simulink subsystem "Joystick_Input_To_Swerve_Drive_sub"  (R2023b)
settings: Solver=VariableStepAuto  StartTime=0.0  StopTime=10.0  RelTol=1e-3
undefined symbols (not defined in the file): AT_XY_Control_Gain, AT_Yaw_Control_Gain, Boost_Trigger_High_Speed, Boost_Trigger_Low_Speed, Steering_Abs_Deadband_Range, Steering_Mod_Drv_in, Steering_Mod_Drv_out, Steering_Mod_Str_Rel_in, Steering_Mod_Str_Rel_out, Steering_Relative_Gain, Steering_Twist_Gain, Translation_Twist_Gain
libraries: simulink x14, hdlsllib x5, Controls_Components_lib x1
settings Model: Creator=ander  LastModifiedBy=FIRSTMentor

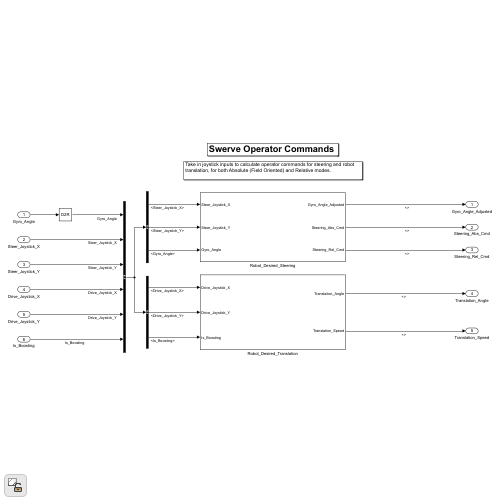
[thumbnail: Simulink's stored preview of the top-level diagram]
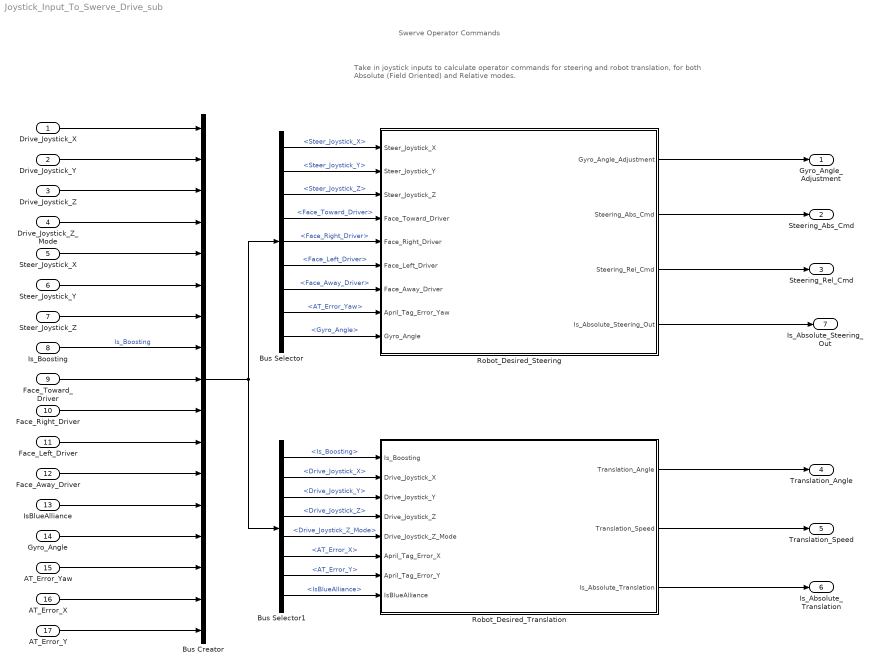
== system Joystick_Input_To_Swerve_Drive_sub ==
  note: Swerve Operator Commands
  note: Take in joystick inputs to calculate operator commands for steering and robot translation, for both Absolute (Field Oriented) and Relative modes.
  Drive_Joystick_X : Inport
  Drive_Joystick_Y : Inport  Port=2
  Drive_Joystick_Z : Inport  Port=3
  Drive_Joystick_Z_Mode : Inport  Port=4
  Steer_Joystick_X : Inport  Port=5
  Steer_Joystick_Y : Inport  Port=6
  Steer_Joystick_Z : Inport  Port=7
  Is_Boosting : Inport  Port=8
  Face_Toward_Driver : Inport  Port=9
  Face_Right_Driver : Inport  Port=10
  Face_Left_Driver : Inport  Port=11
  Face_Away_Driver : Inport  Port=12
  IsBlueAlliance : Inport  Port=13
  Gyro_Angle : Inport  Port=14
  AT_Error_Yaw : Inport  Port=15
  AT_Error_X : Inport  Port=16
  AT_Error_Y : Inport  Port=17
  Bus Creator : BusCreator  Inputs=17
  Bus Selector : BusSelector  OutputSignals=Steer_Joystick_X,Steer_Joystick_Y,Steer_Joystick_Z,Face_Toward_Driver,Face_Right_Driver,Face_Left_Driver,Face_Away_Driver,AT_Error_Yaw,Gyro_Angle
  Bus Selector1 : BusSelector  OutputSignals=Is_Boosting,Drive_Joystick_X,Drive_Joystick_Y,Drive_Joystick_Z,Drive_Joystick_Z_Mode,AT_Error_X,AT_Error_Y,IsBlueAlliance
  Robot_Desired_Steering : Subsystem
  Robot_Desired_Translation : Subsystem
  Gyro_Angle_Adjustment : Outport
  Steering_Abs_Cmd : Outport  Port=2
  Steering_Rel_Cmd : Outport  Port=3
  Translation_Angle : Outport  Port=4
  Translation_Speed : Outport  Port=5
  Is_Absolute_Translation : Outport  Port=6
  Is_Absolute_Steering_Out : Outport  Port=7
  wires:
  Robot_Desired_Steering/4(Is_Absolute_Steering_Out) -> Is_Absolute_Steering_Out/1
  Bus Selector1/5 -> Robot_Desired_Translation/5(Drive_Joystick_Z_Mode)  "<Drive_Joystick_Z_Mode>"
  Drive_Joystick_Z_Mode/1 -> Bus Creator/4
  Bus Selector1/7 -> Robot_Desired_Translation/7(April_Tag_Error_Y)  "<AT_Error_Y>"
  Bus Selector1/6 -> Robot_Desired_Translation/6(April_Tag_Error_X)  "<AT_Error_X>"
  Bus Selector/8 -> Robot_Desired_Steering/8(April_Tag_Error_Yaw)  "<AT_Error_Yaw>"
  Robot_Desired_Translation/3(Is_Absolute_Translation) -> Is_Absolute_Translation/1
  Bus Selector1/4 -> Robot_Desired_Translation/4(Drive_Joystick_Z)  "<Drive_Joystick_Z>"
  Bus Selector1/1 -> Robot_Desired_Translation/1(Is_Boosting)  "<Is_Boosting>"
  Robot_Desired_Steering/3(Steering_Rel_Cmd) -> Steering_Rel_Cmd/1
  Robot_Desired_Steering/2(Steering_Abs_Cmd) -> Steering_Abs_Cmd/1
  Robot_Desired_Steering/1(Gyro_Angle_Adjustment) -> Gyro_Angle_Adjustment/1
  Bus Selector/2 -> Robot_Desired_Steering/2(Steer_Joystick_Y)  "<Steer_Joystick_Y>"
  Bus Selector/1 -> Robot_Desired_Steering/1(Steer_Joystick_X)  "<Steer_Joystick_X>"
  Robot_Desired_Translation/1(Translation_Angle) -> Translation_Angle/1
  Robot_Desired_Translation/2(Translation_Speed) -> Translation_Speed/1
  Bus Creator/1 -> Bus Selector/1, Bus Selector1/1
  Bus Selector1/3 -> Robot_Desired_Translation/3(Drive_Joystick_Y)  "<Drive_Joystick_Y>"
  Bus Selector1/2 -> Robot_Desired_Translation/2(Drive_Joystick_X)  "<Drive_Joystick_X>"
  Drive_Joystick_X/1 -> Bus Creator/1
  Drive_Joystick_Z/1 -> Bus Creator/3
  Steer_Joystick_Y/1 -> Bus Creator/6
  Drive_Joystick_Y/1 -> Bus Creator/2
  Steer_Joystick_X/1 -> Bus Creator/5
  Steer_Joystick_Z/1 -> Bus Creator/7
  Face_Toward_Driver/1 -> Bus Creator/9
  Face_Right_Driver/1 -> Bus Creator/10
  Face_Left_Driver/1 -> Bus Creator/11
  Face_Away_Driver/1 -> Bus Creator/12
  Is_Boosting/1 -> Bus Creator/8  "Is_Boosting"
  Bus Selector/4 -> Robot_Desired_Steering/4(Face_Toward_Driver)  "<Face_Toward_Driver>"
  Bus Selector/3 -> Robot_Desired_Steering/3(Steer_Joystick_Z)  "<Steer_Joystick_Z>"
  Bus Selector/5 -> Robot_Desired_Steering/5(Face_Right_Driver)  "<Face_Right_Driver>"
  Bus Selector/6 -> Robot_Desired_Steering/6(Face_Left_Driver)  "<Face_Left_Driver>"
  Bus Selector/7 -> Robot_Desired_Steering/7(Face_Away_Driver)  "<Face_Away_Driver>"
  IsBlueAlliance/1 -> Bus Creator/13
  AT_Error_Yaw/1 -> Bus Creator/15
  AT_Error_X/1 -> Bus Creator/16
  AT_Error_Y/1 -> Bus Creator/17
  Bus Selector1/8 -> Robot_Desired_Translation/8(IsBlueAlliance)  "<IsBlueAlliance>"
  Gyro_Angle/1 -> Bus Creator/14
  Bus Selector/9 -> Robot_Desired_Steering/9(Gyro_Angle)  "<Gyro_Angle>"

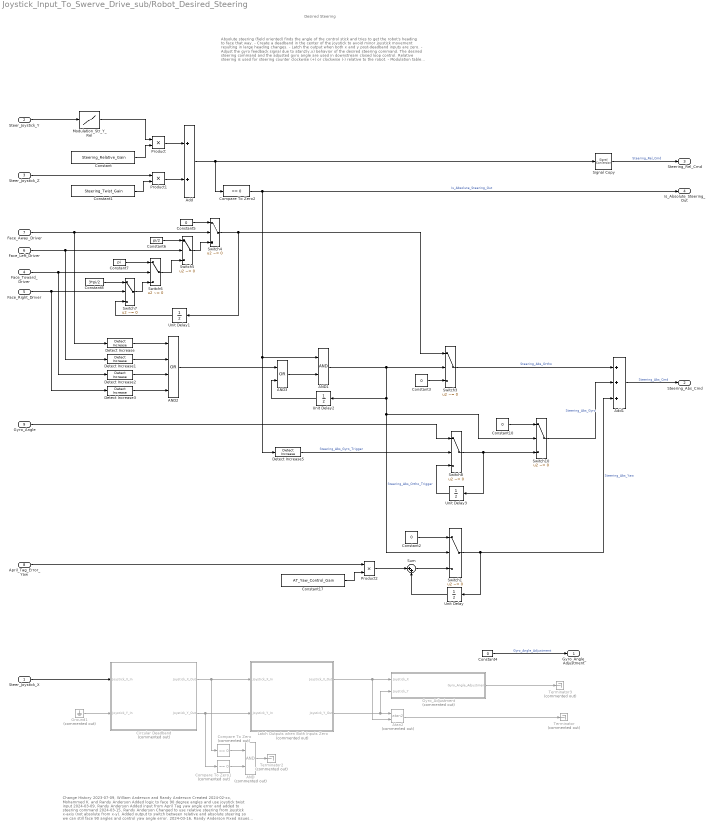
== system Joystick_Input_To_Swerve_Drive_sub/Robot_Desired_Steering ==
  note: Change History
      | 2023-07-09, William Anderson and Randy Anderson
      | Created
      | 2024-02-xx, Mohammed K. and Randy Anderson
      | Added logic to face 90 degree angles and use joystick twist input
      | 2024-03-09, Randy Anderson
      | Added input from April Tag yaw angle error and added to steering command
      | 2024-03-15, Randy Anderson
      | Changed to use relative steering from joystick x-axis (not absolute from x-y).
      | Added output to switch between relative and absolute steering so we can still
      | face 90 angles and control yaw angle error.
      | 2024-03-16, Randy Anderson
      | Fixed issues with using yaw error and snapping to 90 degree angles when
      | coupled with relative steering.
      | 2024-03-18, Randy Anderosn
      | Added gyro angle input to make corrections to robot heading while driving
      | without driver steering input.
  note: Desired Steering
  note: Absolute steering (field oriented) finds the angle of the control stick and tries to get the robot's heading to face that way.
      | - Create a deadband in the center of the joystick to avoid minor joystick movement resulting in large heading changes.
      | - Latch the output when both x and y post-deadband inputs are zero.
      | - Adjust the gyro feedback signal due to atan2(y,x) behavior of the desired steering command. The desired steering command and the adjusted gyro angle are used in downstream closed loop control.
      |
      | Relative steering is used for steering counter clockwise (+) or clockwise (-) relative to the robot.
      | - Modulation table for joystick input. Only one axis of the steering joystck is used.
      | - The gain block adjusts how fast the robot will rotate.
      |
      | NEED TO UPDATE
  Steer_Joystick_X : Inport
  Steer_Joystick_Y : Inport  Port=2
  Steer_Joystick_Z : Inport  Port=3
  Face_Toward_Driver : Inport  Port=4
  Face_Right_Driver : Inport  Port=5
  Face_Left_Driver : Inport  Port=6
  Face_Away_Driver : Inport  Port=7
  April_Tag_Error_Yaw : Inport  Port=8
  Gyro_Angle : Inport  Port=9
  AND : Logic  Commented=on  AllPortsSameDT=off  OutDataTypeStr=boolean
  AND1 : Logic  AllPortsSameDT=off  OutDataTypeStr=boolean
  AND2 : Logic  Operator=OR  Inputs=4  AllPortsSameDT=off  OutDataTypeStr=boolean
  AND3 : Logic  Operator=OR  AllPortsSameDT=off  OutDataTypeStr=boolean
  Add : Sum
  Add1 : Sum  Inputs=3
  Atan2 : Trigonometry  Commented=on  Operator=atan2
  Circular Deadband : Subsystem  Commented=on
  Compare To Zero : simulink/Logic and Bit Operations/Compare To Zero  Commented=on  relop===  OutDataTypeStr=boolean
  Compare To Zero1 : simulink/Logic and Bit Operations/Compare To Zero  Commented=on  relop===  OutDataTypeStr=boolean
  Compare To Zero2 : simulink/Logic and Bit Operations/Compare To Zero  relop===  OutDataTypeStr=boolean
  Constant : Constant  Value=Steering_Relative_Gain
  Constant1 : Constant  Value=Steering_Twist_Gain
  Constant{2..5,10} (5 alike) : Constant  Value=0
  Constant17 : Constant  Value=AT_Yaw_Control_Gain
  Constant6 : Constant  Value=pi/2
  Constant7 : Constant  Value=pi
  Constant8 : Constant  Value=3*pi/2
  Detect Increase{,1..3,5} (5 alike) : simulink/Logic and Bit Operations/Detect Increase  vinit=0.0  OutDataTypeStr=boolean
  Ground1 : Ground  Commented=on
  Gyro_Adjustment : Subsystem  Commented=on
  Latch Outputs when Both Inputs Zero : Subsystem  Commented=on
  Modulation_Str_Y_Rel : Lookup_n-D  NumberOfTableDimensions=1  BreakpointsForDimension1=Steering_Mod_Str_Rel_in  Table=Steering_Mod_Str_Rel_out  ExtrapMethod=Clip  InternalRulePriority=Speed  RndMeth=Simplest
  Product : Product
  Product1 : Product
  Product2 : Product
  Signal Copy : SignalConversion  OverrideOpt=off
  Sum : Sum  Inputs=|++
  Switch{1,3..8,10} (8 alike) : Switch  Criteria=u2 ~= 0  SaturateOnIntegerOverflow=off  InputSameDT=off
  Terminator : Terminator  Commented=on
  Terminator2 : Terminator  Commented=on
  Terminator3 : Terminator  Commented=on
  Unit Delay{,1..3} (4 alike) : UnitDelay  SampleTime=-1  HasFrameUpgradeWarning=on
  Gyro_Angle_Adjustment : Outport
  Steering_Abs_Cmd : Outport  Port=2
  Steering_Rel_Cmd : Outport  Port=3
  Is_Absolute_Steering_Out : Outport  Port=4
  wires:
  Product2/1 -> Sum/1
  Constant2/1 -> Switch1/1
  Unit Delay/1 -> Sum/2
  Sum/1 -> Switch1/3
  Switch10/1 -> Add1/2  "Steering_Abs_Gyro"
  Steer_Joystick_Y/1 -> Modulation_Str_Y_Rel/1
  Detect Increase5/1 -> Switch8/2  "Steering_Abs_Gyro_Trigger"
  Unit Delay3/1 -> Switch8/3
  Switch8/1 -> Unit Delay3/1, Switch10/3
  Gyro_Angle/1 -> Switch8/1
  Switch3/1 -> Add1/1  "Steering_Abs_Ortho"
  Constant3/1 -> Switch3/3
  Add1/1 -> Steering_Abs_Cmd/1  "Steering_Abs_Cmd"
  Product1/1 -> Add/2
  Product/1 -> Add/1
  Steer_Joystick_X/1 -> Circular Deadband/1(Joystick_X_In)
  Ground1/1 -> Circular Deadband/2(Joystick_Y_In)
  Gyro_Adjustment/1(Gyro_Angle_Adjustment) -> Terminator3/1
  Face_Right_Driver/1 -> Detect Increase3/1, Switch7/2
  Face_Toward_Driver/1 -> Detect Increase2/1, Switch6/2
  Face_Left_Driver/1 -> Detect Increase1/1, Switch5/2
  Face_Away_Driver/1 -> Detect Increase/1, Switch4/2
  Switch7/1 -> Switch6/3
  Switch5/1 -> Switch4/3
  Constant8/1 -> Switch7/1
  Constant6/1 -> Switch5/1
  Switch6/1 -> Switch5/3
  Constant7/1 -> Switch6/1
  Constant5/1 -> Switch4/1
  Constant1/1 -> Product1/2
  Switch1/1 -> Add1/3, Unit Delay/1  "Steering_Abs_Yaw"
  Compare To Zero1/1 -> AND/2
  Compare To Zero/1 -> AND/1
  Steer_Joystick_Z/1 -> Product1/1
  Modulation_Str_Y_Rel/1 -> Product/1
  Add/1 -> Compare To Zero2/1, Signal Copy/1
  Constant/1 -> Product/2
  Constant4/1 -> Gyro_Angle_Adjustment/1  "Gyro_Angle_Adjustment"
  Latch Outputs when Both Inputs Zero/2(Joystick_Y_Out) -> Gyro_Adjustment/2(Joystick_Y), Atan2/1
  Circular Deadband/2(Joystick_Y_Out) -> Compare To Zero1/1, Latch Outputs when Both Inputs Zero/2(Joystick_Y_In)
  Circular Deadband/1(Joystick_X_Out) -> Latch Outputs when Both Inputs Zero/1(Joystick_X_In), Compare To Zero/1
  Latch Outputs when Both Inputs Zero/1(Joystick_X_Out) -> Atan2/2, Gyro_Adjustment/1(Joystick_X)
  Switch4/1 -> Unit Delay1/1, Switch3/1
  Unit Delay1/1 -> Switch7/3
  AND1/1 -> Unit Delay2/1, Switch10/2, Switch1/2, Switch3/2  "Steering_Abs_Ortho_Trigger"
  Detect Increase/1 -> AND2/1
  Detect Increase1/1 -> AND2/2
  Detect Increase2/1 -> AND2/3
  Detect Increase3/1 -> AND2/4
  AND2/1 -> AND3/1
  AND3/1 -> AND1/2
  Unit Delay2/1 -> AND3/2
  Constant17/1 -> Product2/2
  April_Tag_Error_Yaw/1 -> Product2/1
  Atan2/1 -> Terminator/1
  Compare To Zero2/1 -> Detect Increase5/1, AND1/1, Is_Absolute_Steering_Out/1  "Is_Absolute_Steering_Out"
  AND/1 -> Terminator2/1
  Signal Copy/1 -> Steering_Rel_Cmd/1  "Steering_Rel_Cmd"
  Constant10/1 -> Switch10/1

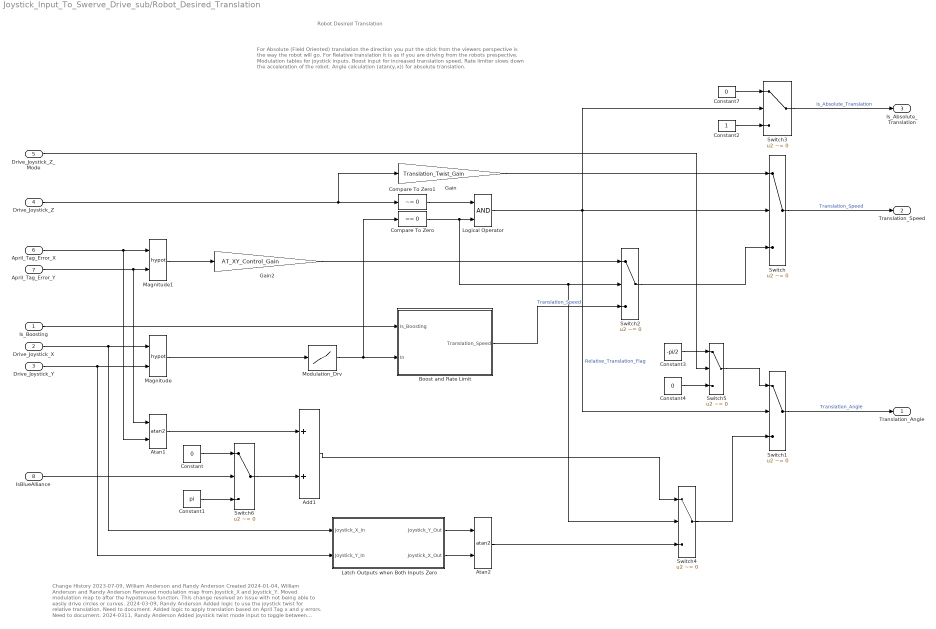
== system Joystick_Input_To_Swerve_Drive_sub/Robot_Desired_Translation ==
  note: Change History
      | 2023-07-09, William Anderson and Randy Anderson
      | Created
      | 2024-01-04, William Anderson and Randy Anderson
      | Removed modulation map from Joystick_X and Joystick_Y.
      | Moved modulation map to after the hypotenuse function.
      | This change resolved an issue with not being able to easily drive circles or curves.
      | 2024-03-09, Randy Anderson
      | Added logic to use the joystick twist for relative translation. Need to document.
      | Added logic to apply translation based on April Tag x and y errors. Need to document.
      | 2024-0311, Randy Anderson
      | Added joystick twist mode input to toggle between fwd/rev and left/right relative translation.
      | 2024-03-20, Randy Anderson
      | Changed from IsRedAlliance to IsBlueAlliance and swapped 0 and pi at the switch.
  note: For Absolute (Field Oriented) translation the direction you put the stick from the viewers perspective is the way the robot will go.
      |
      | For Relative translation it is as if you are driving from the robots prespective.
      |
      | Modulation tables for joystick inputs.
      | Boost input for increased translation speed.
      | Rate limiter slows down the acceleration of the robot.
      | Angle calculation (atan(y,x)) for absolute translation.
  note: Robot Desired Translation
  Is_Boosting : Inport
  Drive_Joystick_X : Inport  Port=2
  Drive_Joystick_Y : Inport  Port=3
  Drive_Joystick_Z : Inport  Port=4
  Drive_Joystick_Z_Mode : Inport  Port=5
  April_Tag_Error_X : Inport  Port=6
  April_Tag_Error_Y : Inport  Port=7
  IsBlueAlliance : Inport  Port=8
  Add1 : Sum
  Atan1 : Trigonometry  Operator=atan2
  Atan2 : Trigonometry  Operator=atan2
  Boost and Rate Limit : Subsystem
  Compare To Zero : simulink/Logic and Bit Operations/Compare To Zero  relop===  OutDataTypeStr=boolean
  Compare To Zero1 : simulink/Logic and Bit Operations/Compare To Zero  relop=~=  OutDataTypeStr=boolean
  Constant : Constant  Value=0
  Constant1 : Constant  Value=pi
  Constant2 : Constant  OutDataTypeStr=Inherit: Inherit via back propagation
  Constant3 : Constant  Value=-pi/2
  Constant4 : Constant  Value=0
  Constant7 : Constant  Value=0  OutDataTypeStr=Inherit: Inherit via back propagation
  Gain : Gain  Gain=Translation_Twist_Gain
  Gain2 : Gain  Gain=AT_XY_Control_Gain
  Latch Outputs when Both Inputs Zero : Subsystem
  Logical Operator : Logic  AllPortsSameDT=off  OutDataTypeStr=boolean
  Magnitude : Math  Operator=hypot
  Magnitude1 : Math  Operator=hypot
  Modulation_Drv : Lookup_n-D  NumberOfTableDimensions=1  BreakpointsForDimension1=Steering_Mod_Drv_in  Table=Steering_Mod_Drv_out  ExtrapMethod=Clip  InternalRulePriority=Speed  RndMeth=Simplest
  Switch{,1..6} (7 alike) : Switch  Criteria=u2 ~= 0  SaturateOnIntegerOverflow=off  InputSameDT=off
  Translation_Angle : Outport
  Translation_Speed : Outport  Port=2
  Is_Absolute_Translation : Outport  Port=3
  wires:
  Atan1/1 -> Add1/1
  Constant/1 -> Switch6/1
  Constant1/1 -> Switch6/3
  Switch6/1 -> Add1/2
  IsBlueAlliance/1 -> Switch6/2
  Add1/1 -> Switch4/1
  Modulation_Drv/1 -> Boost and Rate Limit/2(In), Compare To Zero/1
  Drive_Joystick_Y/1 -> Magnitude/2, Latch Outputs when Both Inputs Zero/2(Joystick_Y_In)
  Drive_Joystick_X/1 -> Magnitude/1, Latch Outputs when Both Inputs Zero/1(Joystick_X_In)
  Magnitude/1 -> Modulation_Drv/1
  Switch1/1 -> Translation_Angle/1  "Translation_Angle"
  Switch/1 -> Translation_Speed/1  "Translation_Speed"
  Is_Boosting/1 -> Boost and Rate Limit/1(Is_Boosting)
  Latch Outputs when Both Inputs Zero/2(Joystick_X_Out) -> Atan2/2
  Latch Outputs when Both Inputs Zero/1(Joystick_Y_Out) -> Atan2/1
  Drive_Joystick_Z/1 -> Gain/1, Compare To Zero1/1
  Logical Operator/1 -> Switch/2, Switch1/2, Switch3/2  "Relative_Translation_Flag"
  Compare To Zero1/1 -> Logical Operator/1
  Compare To Zero/1 -> Switch4/2, Switch2/2, Logical Operator/2
  Gain/1 -> Switch/1
  Constant2/1 -> Switch3/3
  Constant7/1 -> Switch3/1
  Switch3/1 -> Is_Absolute_Translation/1  "Is_Absolute_Translation"
  Switch2/1 -> Switch/3
  Boost and Rate Limit/1(Translation_Speed) -> Switch2/3  "Translation_Speed"
  April_Tag_Error_X/1 -> Atan1/2, Magnitude1/1
  April_Tag_Error_Y/1 -> Magnitude1/2, Atan1/1
  Magnitude1/1 -> Gain2/1
  Atan2/1 -> Switch4/3
  Switch4/1 -> Switch1/3
  Gain2/1 -> Switch2/1
  Switch5/1 -> Switch1/1
  Constant3/1 -> Switch5/1
  Drive_Joystick_Z_Mode/1 -> Switch5/2
  Constant4/1 -> Switch5/3

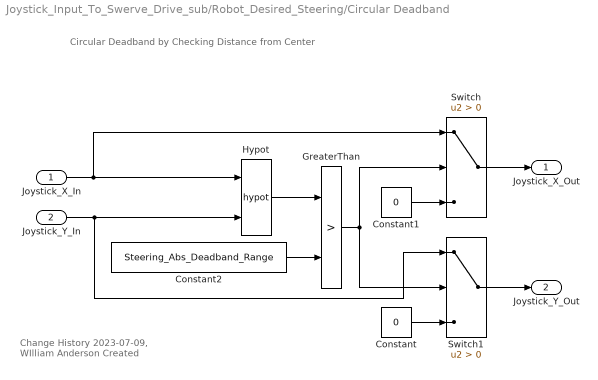
== system Joystick_Input_To_Swerve_Drive_sub/Robot_Desired_Steering/Circular Deadband ==
  note: Change History
      | 2023-07-09, WIlliam Anderson
      | Created
  note: Circular Deadband by Checking Distance from Center
  Joystick_X_In : Inport
  Joystick_Y_In : Inport  Port=2
  Constant : Constant  Value=0
  Constant1 : Constant  Value=0
  Constant2 : Constant  Value=Steering_Abs_Deadband_Range
  GreaterThan : RelationalOperator  Operator=>  OutDataTypeStr=boolean  RndMeth=Simplest  InputSameDT=off
  Hypot : Math  Operator=hypot
  Switch : Switch  Criteria=u2 > Threshold  SaturateOnIntegerOverflow=off  InputSameDT=off
  Switch1 : Switch  Criteria=u2 > Threshold  SaturateOnIntegerOverflow=off  InputSameDT=off
  Joystick_X_Out : Outport
  Joystick_Y_Out : Outport  Port=2
  wires:
  Switch1/1 -> Joystick_Y_Out/1
  Switch/1 -> Joystick_X_Out/1
  Constant/1 -> Switch1/3
  Constant1/1 -> Switch/3
  Joystick_X_In/1 -> Hypot/1, Switch/1
  Joystick_Y_In/1 -> Switch1/1, Hypot/2
  Hypot/1 -> GreaterThan/1
  Constant2/1 -> GreaterThan/2
  GreaterThan/1 -> Switch/2, Switch1/2

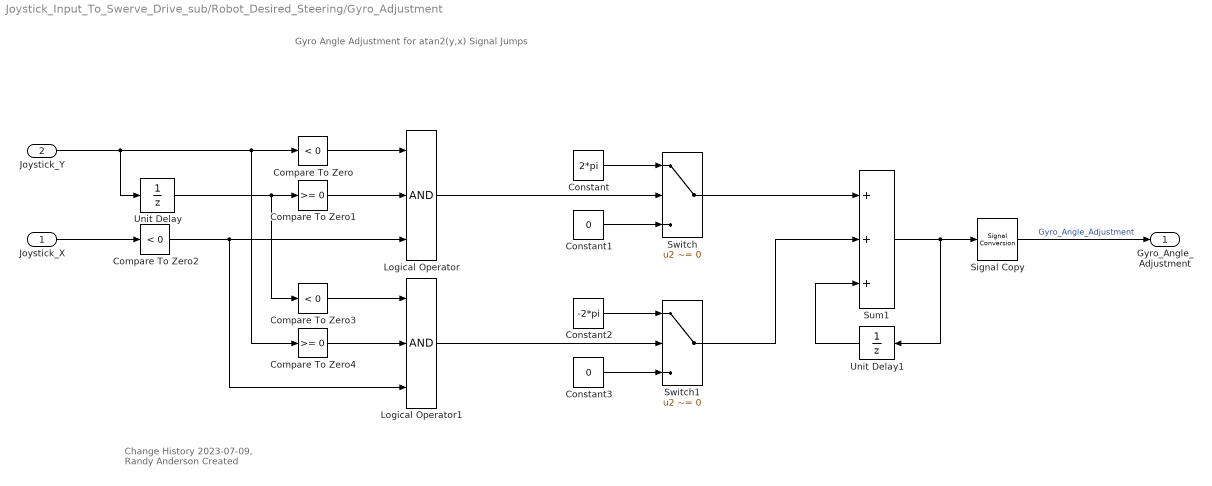
== system Joystick_Input_To_Swerve_Drive_sub/Robot_Desired_Steering/Gyro_Adjustment ==
  note: Change History
      | 2023-07-09, Randy Anderson
      | Created
  note: Gyro Angle Adjustment for atan2(y,x) Signal Jumps
  Joystick_X : Inport
  Joystick_Y : Inport  Port=2
  Compare To Zero : hdlsllib/Logic and Bit Operations/Compare To Zero  relop=<  OutDataTypeStr=boolean
  Compare To Zero1 : hdlsllib/Logic and Bit Operations/Compare To Zero  relop=>=  OutDataTypeStr=boolean
  Compare To Zero2 : hdlsllib/Logic and Bit Operations/Compare To Zero  relop=<  OutDataTypeStr=boolean
  Compare To Zero3 : hdlsllib/Logic and Bit Operations/Compare To Zero  relop=<  OutDataTypeStr=boolean
  Compare To Zero4 : hdlsllib/Logic and Bit Operations/Compare To Zero  relop=>=  OutDataTypeStr=boolean
  Constant : Constant  Value=2*pi
  Constant1 : Constant  Value=0
  Constant2 : Constant  Value=-2*pi
  Constant3 : Constant  Value=0
  Logical Operator : Logic  Inputs=3  AllPortsSameDT=off  OutDataTypeStr=boolean
  Logical Operator1 : Logic  Inputs=3  AllPortsSameDT=off  OutDataTypeStr=boolean
  Signal Copy : SignalConversion  OverrideOpt=off
  Sum1 : Sum  Inputs=3
  Switch : Switch  Criteria=u2 ~= 0  SaturateOnIntegerOverflow=off  InputSameDT=off
  Switch1 : Switch  Criteria=u2 ~= 0  SaturateOnIntegerOverflow=off  InputSameDT=off
  Unit Delay : UnitDelay  SampleTime=-1  HasFrameUpgradeWarning=on
  Unit Delay1 : UnitDelay  SampleTime=-1  HasFrameUpgradeWarning=on
  Gyro_Angle_Adjustment : Outport
  wires:
  Signal Copy/1 -> Gyro_Angle_Adjustment/1  "Gyro_Angle_Adjustment"
  Switch1/1 -> Sum1/2
  Constant2/1 -> Switch1/1
  Constant3/1 -> Switch1/3
  Logical Operator1/1 -> Switch1/2
  Compare To Zero4/1 -> Logical Operator1/2
  Compare To Zero3/1 -> Logical Operator1/1
  Compare To Zero2/1 -> Logical Operator/3, Logical Operator1/3
  Joystick_X/1 -> Compare To Zero2/1
  Unit Delay1/1 -> Sum1/3
  Switch/1 -> Sum1/1
  Sum1/1 -> Signal Copy/1, Unit Delay1/1
  Logical Operator/1 -> Switch/2
  Constant1/1 -> Switch/3
  Constant/1 -> Switch/1
  Compare To Zero1/1 -> Logical Operator/2
  Compare To Zero/1 -> Logical Operator/1
  Unit Delay/1 -> Compare To Zero1/1, Compare To Zero3/1
  Joystick_Y/1 -> Unit Delay/1, Compare To Zero/1, Compare To Zero4/1

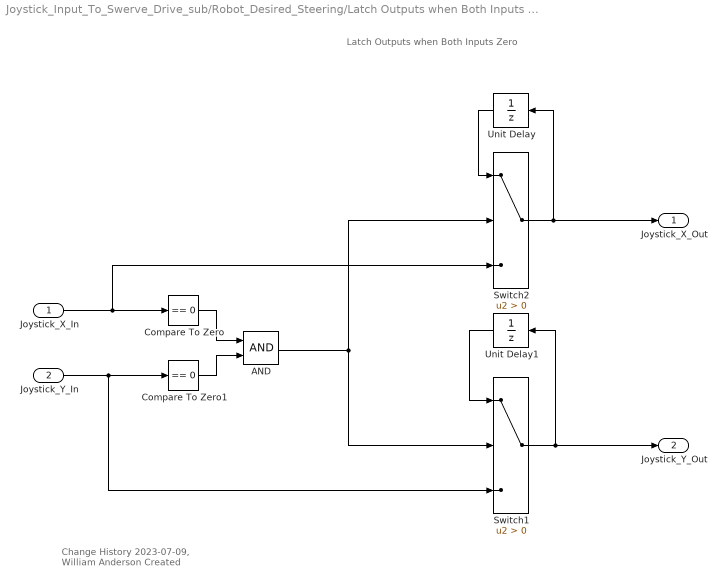
== system Joystick_Input_To_Swerve_Drive_sub/Robot_Desired_Steering/Latch Outputs when Both Inputs Zero ==
  note: Change History
      | 2023-07-09, William Anderson
      | Created
  note: Latch Outputs when Both Inputs Zero
  Joystick_X_In : Inport
  Joystick_Y_In : Inport  Port=2
  AND : Logic  AllPortsSameDT=off  OutDataTypeStr=boolean
  Compare To Zero : simulink/Logic and Bit Operations/Compare To Zero  relop===  OutDataTypeStr=boolean
  Compare To Zero1 : simulink/Logic and Bit Operations/Compare To Zero  relop===  OutDataTypeStr=boolean
  Switch1 : Switch  Criteria=u2 > Threshold  SaturateOnIntegerOverflow=off  InputSameDT=off
  Switch2 : Switch  Criteria=u2 > Threshold  SaturateOnIntegerOverflow=off  InputSameDT=off
  Unit Delay : UnitDelay  SampleTime=-1  HasFrameUpgradeWarning=on
  Unit Delay1 : UnitDelay  SampleTime=-1  HasFrameUpgradeWarning=on
  Joystick_X_Out : Outport
  Joystick_Y_Out : Outport  Port=2
  wires:
  Switch1/1 -> Joystick_Y_Out/1, Unit Delay1/1
  Switch2/1 -> Joystick_X_Out/1, Unit Delay/1
  Joystick_X_In/1 -> Switch2/3, Compare To Zero/1
  Joystick_Y_In/1 -> Switch1/3, Compare To Zero1/1
  Compare To Zero1/1 -> AND/2
  Compare To Zero/1 -> AND/1
  AND/1 -> Switch1/2, Switch2/2
  Unit Delay/1 -> Switch2/1
  Unit Delay1/1 -> Switch1/1

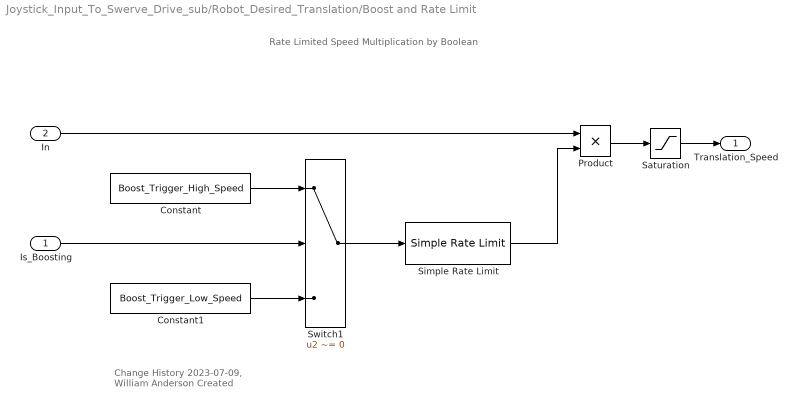
== system Joystick_Input_To_Swerve_Drive_sub/Robot_Desired_Translation/Boost and Rate Limit ==
  note: Change History
      | 2023-07-09, William Anderson
      | Created
  note: Rate Limited Speed Multiplication by Boolean
  Is_Boosting : Inport
  In : Inport  Port=2
  Constant : Constant  Value=Boost_Trigger_High_Speed
  Constant1 : Constant  Value=Boost_Trigger_Low_Speed
  Product : Product
  Saturation : Saturate  UpperLimit=Boost_Trigger_High_Speed  LowerLimit=-Boost_Trigger_High_Speed
  Simple Rate Limit : Controls_Components_lib/Simple Rate Limit  Rate_Limit_Inc=Boost_Trigger_Increasing_Limit  Rate_Limit_Dec=Boost_Trigger_Decreasing_Limit
  Switch1 : Switch  Criteria=u2 ~= 0  SaturateOnIntegerOverflow=off  InputSameDT=off
  Translation_Speed : Outport
  wires:
  Is_Boosting/1 -> Switch1/2
  Constant/1 -> Switch1/1
  Constant1/1 -> Switch1/3
  Switch1/1 -> Simple Rate Limit/1
  In/1 -> Product/1
  Product/1 -> Saturation/1
  Simple Rate Limit/1 -> Product/2
  Saturation/1 -> Translation_Speed/1

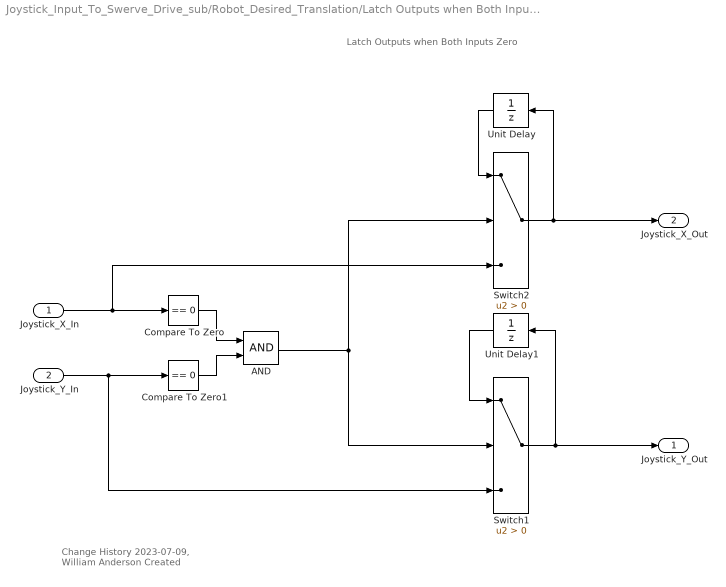
== system Joystick_Input_To_Swerve_Drive_sub/Robot_Desired_Translation/Latch Outputs when Both Inputs Zero ==
  note: Change History
      | 2023-07-09, William Anderson
      | Created
  note: Latch Outputs when Both Inputs Zero
  Joystick_X_In : Inport
  Joystick_Y_In : Inport  Port=2
  AND : Logic  AllPortsSameDT=off  OutDataTypeStr=boolean
  Compare To Zero : simulink/Logic and Bit Operations/Compare To Zero  relop===  OutDataTypeStr=boolean
  Compare To Zero1 : simulink/Logic and Bit Operations/Compare To Zero  relop===  OutDataTypeStr=boolean
  Switch1 : Switch  Criteria=u2 > Threshold  SaturateOnIntegerOverflow=off  InputSameDT=off
  Switch2 : Switch  Criteria=u2 > Threshold  SaturateOnIntegerOverflow=off  InputSameDT=off
  Unit Delay : UnitDelay  SampleTime=-1  HasFrameUpgradeWarning=on
  Unit Delay1 : UnitDelay  SampleTime=-1  HasFrameUpgradeWarning=on
  Joystick_Y_Out : Outport
  Joystick_X_Out : Outport  Port=2
  wires:
  Switch1/1 -> Joystick_Y_Out/1, Unit Delay1/1
  Switch2/1 -> Joystick_X_Out/1, Unit Delay/1
  Joystick_X_In/1 -> Switch2/3, Compare To Zero/1
  Joystick_Y_In/1 -> Switch1/3, Compare To Zero1/1
  Compare To Zero1/1 -> AND/2
  Compare To Zero/1 -> AND/1
  AND/1 -> Switch1/2, Switch2/2
  Unit Delay/1 -> Switch2/1
  Unit Delay1/1 -> Switch1/1
